simulink model "SimulateDroneTracking"  (R2025b)
settings: Solver=VariableStepAuto  StartTime=0.0  StopTime=5  RelTol=1e-3
undefined symbols (not defined in the file or in its folder): Sim3dSensor
libraries: sim3dcameralib x1, sim3dlib x1, uavsim3dlib x1
settings Model: Creator=ryder  LastModifiedBy=ryder

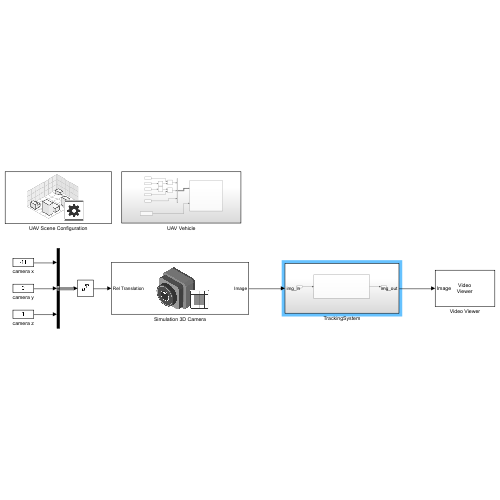
[thumbnail: Simulink's stored preview of the top-level diagram]
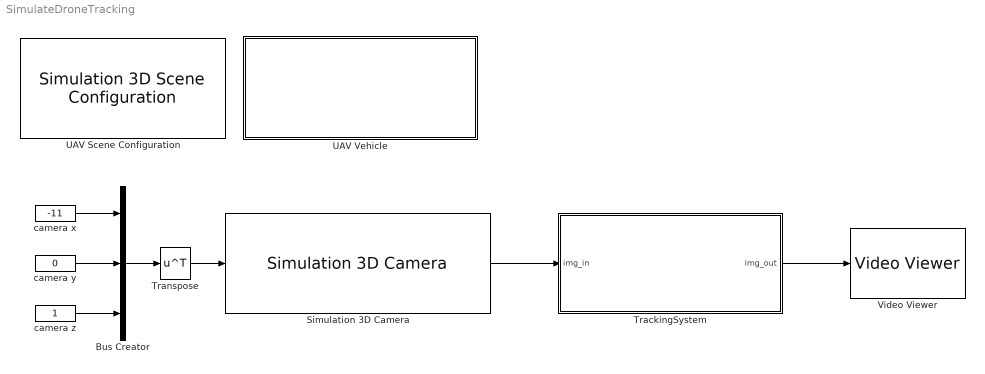
== system SimulateDroneTracking ==
  Bus Creator : BusCreator  Inputs=3
  Simulation 3D Camera : sim3dcameralib/Simulation 3D Camera  Priority=1  sensorTag=Sim3dSensor�  sensorId=1  sensorName=Sim3dSensor�  vehTagList={'DefaultQuadcopter';'Scene Origin'}  vehTag=Scene Origin  CoordinateSystem=ISO8855  mountLoc=Origin  offsetFlag=on  tmountOffset=[0, 0, 0]  extTmount=on  rmountOffset=[0, 0, 0]  extRmount=off  FocalLength=[1109, 1109]  OpticalCenter=[640, 360]  ImageSize=[720,1280]  RadialDistortion=[0, 0]  TangentialDistortion=[0, 0]  SensorSkew=0  VisualizeFieldOfView=off  FieldOfViewRange=61  DepthOutportEnabled=off  SemanticOutportEnabled=off  TransformOutportEnabled=off  SampleTime=-1  mountPoint=[0 0 0]  mountOrientation=[0 0 0]  aMode=4  ID=1
      settings: LibrarySourceBlock=uavsim3dlib/Simulation 3D Camera
  TrackingSystem : Subsystem
  Transpose : Math  Operator=transpose
  UAV Scene Configuration : sim3dlib/Simulation 3D Scene Configuration  Priority=0  ProjectFormat=Default Scenes  SceneDesc=Airport  ProjectName=C:\Program Files\MATLAB\R2025b\toolbox\shared\sim3d_projects\automotive_project_windows\UE\WindowsNoEditor\VehicleSimulation.exe  ScenePath=/Game/Maps/USCityBlock  EnableOpenDRIVE=off  vehTagList={'Custom';'DefaultQuadcopter';'Scene Origin'}  vehTag=DefaultQuadcopter  AttachedCameraRelativeTranslation=[0 0 0]  FreeCameraDefaultInitialTranslation=[-6, 0, 2]  AttachedCameraRelativeRotation=[0 0 0]  FreeCameraDefaultInitialRotation=[0, -15, 0]  ViewpointName=Custom  FreeCameraInitialTranslation=[0, 0, 0]  ViewpointTranslation=[0, 0, 0]  FreeCameraInitialRotation=[0, 0, 0]  ViewpointRotation=[0, 0, 0]  OpVisEn=off  Ts=1/60  EnableWindow=off  EnableRemoteAccess=off  EnableWeather=off  SunAzimuth=90  SunAltitude=40.0  EnableGeospatialSun=off  Latitude=0  Longitude=0  Date=2023-01-01  Time=10:30:00  GeoTimeZone=-5.0  SunDaylightSaving=off  wind=1  clouds=10  EnableVolumetricClouds=off  CloudCoverage=0  CloudAltitude=6  fog=0  rain=0  RaindropsEffect=off  SnowDensity=0  EnableGeospatial=off  TilesetSource=Earth terrain  UseTrueOrigin=off  OriginHeight=200  OriginLatitude=40.744652  OriginLongitude=-73.988864  MapStyle=Aerial  AdditionalAssetIDs=[]  UseAdvancedSunSky=off  SolarTime=11  TimeZone=-5  Day=21  Month=9  Year=2022  UseDaylightSavingTime=on  DSTStartDay=10  DSTStartMonth=3  DSTEndDay=3  DSTEndMonth=11  DSTSwitchHour=2  sensorTag=MainCamera2  sensorId=2  sensorName=MainCamera2  mountLoc=Origin  offsetFlag=off  tmountOffset=[0, 0, 0]  rmountOffset=[0, 0, 0]  HorizontalResolution=1280  VerticalResolution=720  HorizontalFOV=60  mountPoint=[0 0 0]  mountOrientation=[0 0 0]  aMode=4  ID=2  GeoTrigger=Inactive  ViewNameList={'Custom'}  ViewTranslationList={'[0 0 0]'}  ViewRotationList={'[0 0 0]'}
      settings: LibrarySourceBlock=uavsim3dlib/Simulation 3D Scene Configuration
  UAV Vehicle : Subsystem
  Video Viewer : VideoViewer  FigPos=[835 516 418 304]
  camera x : Constant  Value=-11
  camera y : Constant  Value=0
  camera z : Constant
  wires:
  Simulation 3D Camera/1 -> TrackingSystem/1(img_in)
  camera z/1 -> Bus Creator/3
  camera x/1 -> Bus Creator/1
  camera y/1 -> Bus Creator/2
  Bus Creator/1 -> Transpose/1
  Transpose/1 -> Simulation 3D Camera/1
  TrackingSystem/1(img_out) -> Video Viewer/1

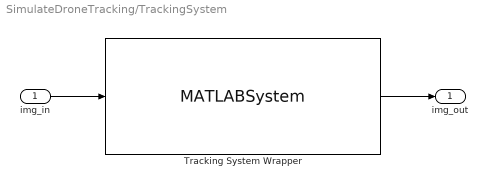
== system SimulateDroneTracking/TrackingSystem ==
  img_in : Inport
  Tracking System Wrapper : MATLABSystem  System=TrackingSystem  TextPrompt=drone  WindowSize=16  RstIntervalMult=16  BbCheckMult=8  MaxImgSize=800  SimulateUsing=Interpreted execution
      mask Type: TrackingSystem
  img_out : Outport
  wires:
  img_in/1 -> Tracking System Wrapper/1
  Tracking System Wrapper/1 -> img_out/1

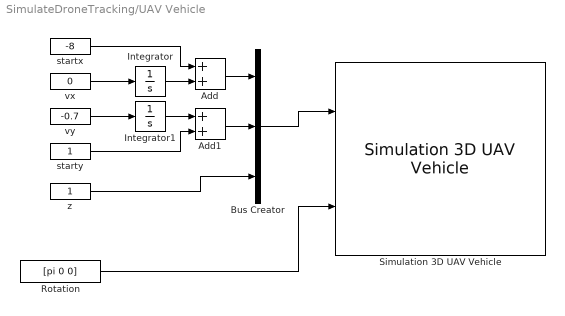
== system SimulateDroneTracking/UAV Vehicle ==
  Add : Sum
  Add1 : Sum
  Bus Creator : BusCreator  Inputs=3
  Integrator : Integrator
  Integrator1 : Integrator
  Rotation : Constant  Value=[pi 0 0]
  Simulation 3D UAV Vehicle : uavsim3dlib/Simulation 3D UAV Vehicle  Priority=-1  Mesh=Quadrotor  MeshPath=/MathWorksUAVContent/UAVs/HexaRotorUAV/HexaRotor.HexaRotor  Color=Black  ActorName=DefaultQuadcopter  UseGlobalFrame=off  InitialTranslation=[0 0 0]  InitialRotation=[0 0 0]  InitialTranslationGlobal=[0 0 0]  InitialGeoOrigin=[0 0 0]  InitialRotationGlobal=[0 0 0]  SampleTime=-1  ActorType=SimulinkVehicle  ID=C  aMode=4  ActorTag=DefaultQuadcopter
  startx : Constant  Value=-8
  starty : Constant
  vx : Constant  Value=0
  vy : Constant  Value=-0.7
  z : Constant
  wires:
  Rotation/1 -> Simulation 3D UAV Vehicle/2
  vy/1 -> Integrator1/1
  vx/1 -> Integrator/1
  startx/1 -> Add/1
  Integrator/1 -> Add/2
  Integrator1/1 -> Add1/1
  starty/1 -> Add1/2
  Add/1 -> Bus Creator/1
  Add1/1 -> Bus Creator/2
  z/1 -> Bus Creator/3
  Bus Creator/1 -> Simulation 3D UAV Vehicle/1
